simulink model "ex2"  (Simulink 6.3)
settings: Solver=ode45  StartTime=0.0  StopTime=10000  MaxStep=1/(100*SymbolRate)  RelTol=1e-3
values from neighbouring files (symbols this model uses):
  SymbolRate = 1000    [ex11.m]    (also in ex2sim.m = 2; ex4sim.m = 2; ex7sim.m = 2)
libraries: commutil2 x4, commsink2 x2, dspbuff3 x2, commdigbbndam2 x2, commchan3 x1, commfilt2 x1, commrandsrc2 x1
settings Model: LastModifiedBy=lxy  StrictBusMsg=None
settings OptimizationCC: InlineInvariantSignals=on

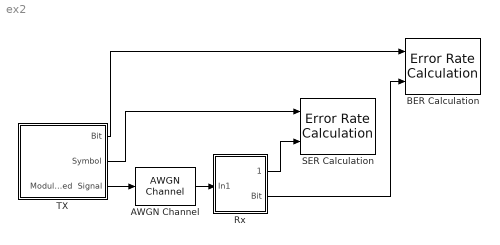
== system ex2 ==
  AWGN Channel : commchan3/AWGN Channel  seed=1111  noiseMode="Signal to noise ratio  (Es/No)"  EbNodB=10  EsNodB=SNR  SNRdB=10  bitsPerSym=1  Ps=5  Tsym=1/SymbolRate  variance=1
  BER Calculation : commsink2/Error Rate Calculation  N=0  st_delay=2*SymbolRate  cp_mode=Entire frame  subframe=[]  PMode=Workspace  WsName=BER  RsMode2=off  stop=off  numErr=100  maxBits=1e6
  Rx : Subsystem
  SER Calculation : commsink2/Error Rate Calculation  N=0  st_delay=SymbolRate  cp_mode=Entire frame  subframe=[]  PMode=Workspace  WsName=SER  RsMode2=off  stop=off  numErr=100  maxBits=1e6
  TX : Subsystem
  wires:
  TX/3(Modulated  Signal) -> AWGN Channel/1
  TX/2(Symbol) -> SER Calculation/1
  Rx/1(Symbol) -> SER Calculation/2
  Rx/2(Bit) -> BER Calculation/2
  TX/1(Bit) -> BER Calculation/1
  AWGN Channel/1 -> Rx/1(In1)

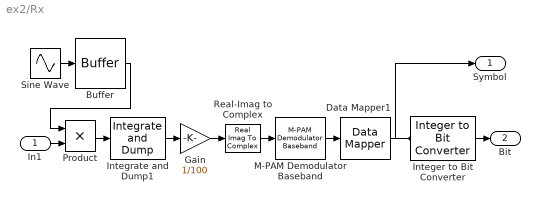
== system ex2/Rx ==
  In1 : Inport
  Buffer : dspbuff3/Buffer  N=100*SymbolRate  V=0  ic=0
  Data Mapper1 : commutil2/Data Mapper  MapMode=Gray to Binary  M=4  MapVec=[0 1 3 2 7 6 4 5]
  Gain : Gain  Gain=1/100
  Integer to Bit Converter : commutil2/Integer to Bit Converter  nbits=2  outDtype=Same as input
  Integrate and Dump1 : commfilt2/Integrate and Dump  obssamples=100  offsetsamples=0  nodump=off
  M-PAM Demodulator Baseband : commdigbbndam2/M-PAM Demodulator Baseband  M=4  OutType=Integer  Dec=Binary  PowType=Min. distance between symbols  MinDist=2  AvgPow=1  PeakPow=1  numSamp=1
  Product : Product  OutDataTypeMode=double  RndMeth=Zero
  Real-Imag to Complex : RealImagToComplex  Input=Real
  Sine Wave : Sin  Amplitude=sqrt(2)  Frequency=2*pi*SymbolRate  Phase=pi/2  Samples=100  SampleTime=1/(100*SymbolRate)
  Symbol : Outport
  Bit : Outport  Port=2
  wires:
  Integer to Bit Converter/1 -> Bit/1
  M-PAM Demodulator Baseband/1 -> Data Mapper1/1
  Real-Imag to Complex/1 -> M-PAM Demodulator Baseband/1
  Integrate and Dump1/1 -> Gain/1
  Gain/1 -> Real-Imag to Complex/1
  Product/1 -> Integrate and Dump1/1
  Sine Wave/1 -> Buffer/1
  Buffer/1 -> Product/1
  In1/1 -> Product/2
  Data Mapper1/1 -> Symbol/1, Integer to Bit Converter/1

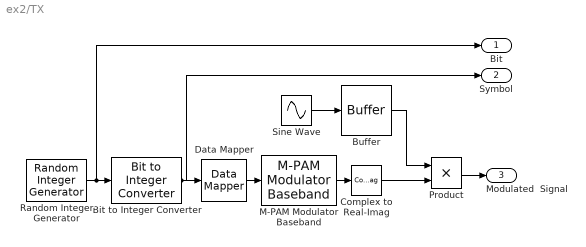
== system ex2/TX ==
  Bit to Integer Converter : commutil2/Bit to Integer Converter  nbits=2  outDtype=Same as input
  Buffer : dspbuff3/Buffer  N=100*SymbolRate  V=0  ic=0
  Complex to Real-Imag : ComplexToRealImag  Output=Real
  Data Mapper : commutil2/Data Mapper  MapMode=Binary to Gray  M=4  MapVec=[0 1 3 2 7 6 4 5]
  M-PAM Modulator Baseband : commdigbbndam2/M-PAM Modulator Baseband  M=4  InType=Integer  Enc=Binary  PowType=Min. distance between symbols  MinDist=2  AvgPow=1  PeakPow=1  numSamp=100
  Product : Product  RndMeth=Zero
  Random Integer Generator : commrandsrc2/Random Integer Generator  mul=2  seed=37  Ts=1/(2*SymbolRate)  frameBased=on  sampPerFrame=2*SymbolRate  orient=off  outDataType=double
  Sine Wave : Sin  Amplitude=sqrt(2)  Frequency=2*pi*SymbolRate  Phase=pi/2  Samples=100  SampleTime=1/(100*SymbolRate)
  Bit : Outport
  Symbol : Outport  Port=2
  Modulated  Signal : Outport  Port=3
  wires:
  Data Mapper/1 -> M-PAM Modulator Baseband/1
  Bit to Integer Converter/1 -> Data Mapper/1, Symbol/1
  Random Integer Generator/1 -> Bit to Integer Converter/1, Bit/1
  M-PAM Modulator Baseband/1 -> Complex to Real-Imag/1
  Complex to Real-Imag/1 -> Product/2
  Sine Wave/1 -> Buffer/1
  Buffer/1 -> Product/1
  Product/1 -> Modulated  Signal/1
